simulink model "f_Madgwick"  (R2015a)
settings: Solver=ode4  StartTime=0.0  StopTime=t(len)  FixedStep=1/freq  RelTol=1e-3
InitFcn:
  | clear all
  | clc
  | 
  | RAW = dlmread('manual_6_raw_16-12.txt');
  | 
  | acc = 1/1000*[RAW(:,1) RAW(:,2) RAW(:,3)]';
  | gyro = 1/1000*[RAW(:,4) RAW(:,5) RAW(:,6)]';
  | mag = [RAW(:,7) RAW(:,8) RAW(:,9)]';
  | 
  | freq = 50; %[Hz] Sampling frequency
  | len = length(RAW);
  | 
  | t = 0 : 1/freq : (len-1)/freq;
StopFcn:
  | close all
  | clc
  | %%
  | 
  | Rm = yout(:,1);
  | Pm = yout(:,2);
  | Ym = yout(:,3);
  | 
  | Rq = yout(:,4);
  | Pq = yout(:,5);
  | Yq = yout(:,6);
  | 
  | Rmu = unwrap(Rm);
  | Pmu = unwrap(Pm);
  | Ymu = unwrap(Ym);
  | 
  | Rqu = unwrap(Rq);
  | Pqu = unwrap(Pq);
  | Yqu = unwrap(Yq);
  | 
  | %% Plotting Roll, Pitch and Yaw angles
  | 
  | figure
  | subplot(3,1,1)
  | plot(tout,Rmu, tout, Rqu)
  | title('Roll')
  | ylabel('[deg]')
  | xlabel('[sec]')
  | legend('Rmu','Rqu')
  | subplot(3,1,2)
  | plot(tout,Pmu, tout, Pqu)
  | title('Pitch')
  | ylabel('[deg]')
  | xlabel('[sec]')
  | legend('Pmu','Pqu')
  | subplot(3,1,3)
  | plot(tout,Ymu, tout, Yqu)
  | title('Yaw')
  | ylabel('[deg]')
  | xlabel('[sec]')
  | legend('Ymu','Yqu')
libraries: aerolibutil x2, aerolibtransform2 x2, dspmathops x1
settings Model: CovSFcnEnable=off  Creator=Mattia  LastModifiedBy=pela
settings DataIOCC: ExternalInput=[t u]
settings DebuggingCC: SolverPrmCheckMsg=warning

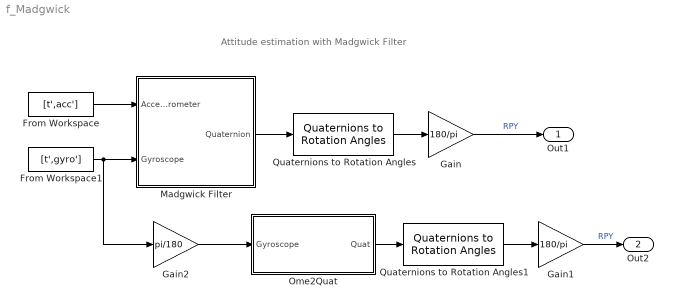
== system f_Madgwick ==
  note: Attitude estimation with Madgwick Filter
  From Workspace : FromWorkspace  VariableName=[t',acc']  SampleTime=0  OutputAfterFinalValue=Setting to zero
  From Workspace1 : FromWorkspace  VariableName=[t',gyro']  SampleTime=0  OutputAfterFinalValue=Setting to zero
  Gain : Gain  Gain=180/pi
  Gain1 : Gain  Gain=180/pi
  Gain2 : Gain  Gain=pi/180
  Madgwick Filter : Subsystem  mask{QUAT0_MF=[1 0 0 0]', beta=0*0.001}
      mask prompts: QUAT0_MF "Quaternion initial condition"; beta "Filter gain"
      mask Display:
      | port_label('input', 1, 'Accelerometer')
      | port_label('input', 2, 'Gyroscope')
      | port_label('Output', 1, 'Quaternion')
  Ome2Quat : Subsystem  mask{QUAT_0=[1 0 0 0]'}
      mask prompts: QUAT_0 "Initial quaternion"
      mask DialogControl DescTextVar Prompt: Here you can set the initial condition for the quaternion integration.
      mask Display:
      | port_label('input', 1, 'Gyroscope')
      | port_label('output', 1, 'Quaternion')
  Quaternions to Rotation Angles : aerolibtransform2/Quaternions to Rotation Angles  rotationOrder=XYZ
  Quaternions to Rotation Angles1 : aerolibtransform2/Quaternions to Rotation Angles  rotationOrder=XYZ
  Out1 : Outport
  Out2 : Outport  Port=2
  wires:
  Quaternions to Rotation Angles/1 -> Gain/1
  Madgwick Filter/1(Quaternion) -> Quaternions to Rotation Angles/1
  From Workspace/1 -> Madgwick Filter/1(Accelerometer)
  Gain/1 -> Out1/1  "RPY"
  Quaternions to Rotation Angles1/1 -> Gain1/1
  Ome2Quat/1(Quat) -> Quaternions to Rotation Angles1/1
  Gain1/1 -> Out2/1  "RPY"
  Gain2/1 -> Ome2Quat/1("Gyroscope ")
  From Workspace1/1 -> Madgwick Filter/2(Gyroscope), Gain2/1

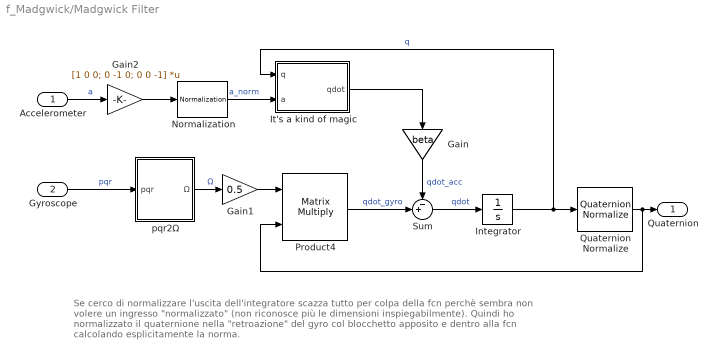
== system f_Madgwick/Madgwick Filter ==
  note: Se cerco di normalizzare l'uscita dell'integratore scazza tutto per colpa della fcn perchè sembra non volere un
      | ingresso "normalizzato" (non riconosce più le dimensioni inspiegabilmente).
      | Quindi ho normalizzato il quaternione nella "retroazione" del gyro col blocchetto apposito e dentro alla fcn calcolando
      | esplicitamente la norma.
  Accelerometer : Inport
  Gyroscope : Inport  Port=2
  Gain : Gain  Gain=beta
  Gain1 : Gain  Gain=0.5
  Gain2 : Gain  Gain=[1 0 0; 0 -1 0; 0 0 -1]  Multiplication=Matrix(K*u)
  Integrator : Integrator  InitialCondition=QUAT0_MF
  It's a kind of magic : MATLAB Function  TreatAsAtomicUnit=on
  Normalization : dspmathops/Normalization  NormType=2-norm  Bias=1e-10  NormOver=Each column  ColComp=on  Dimension=1  outputDataTypeStr=Inherit: Same as product output  outputLastDataTypeStr=Inherit: Same as product output  outputMin=[]  outputMax=[]  accumDataTypeStr=Inherit: Same as product output  accumLastDataTypeStr=Inherit: Same as product output  roundingMode=Floor  overflowMode=off
  Product4 : Product  Multiplication=Matrix(*)
  Quaternion Normalize : aerolibutil/Quaternion Normalize
  Sum : Sum  Inputs=-+|
  pqr2Ω : Subsystem
  Quaternion : Outport
  wires:
  Gyroscope/1 -> pqr2Ω/1(" pqr")  "pqr"
  Gain1/1 -> Product4/1
  pqr2Ω/1(Ω) -> Gain1/1  "Ω"
  Quaternion Normalize/1 -> Quaternion/1, Product4/2
  It's a kind of magic/1(qdot) -> Gain/1
  Normalization/1 -> It's a kind of magic/2(a)  "a_norm"
  Sum/1 -> Integrator/1  "qdot"
  Product4/1 -> Sum/2  "qdot_gyro"
  Integrator/1 -> Quaternion Normalize/1, It's a kind of magic/1(q)  "q"
  Gain/1 -> Sum/1  "qdot_acc"
  Accelerometer/1 -> Gain2/1  "a"
  Gain2/1 -> Normalization/1

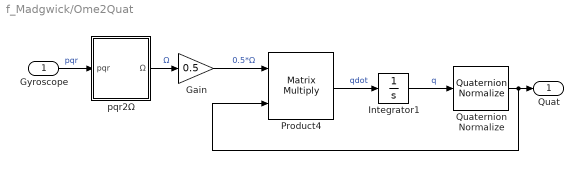
== system f_Madgwick/Ome2Quat ==
  "Gyroscope " : Inport
  Gain : Gain  Gain=0.5
  Integrator1 : Integrator  InitialCondition=QUAT_0
  Product4 : Product  Multiplication=Matrix(*)
  Quaternion Normalize : aerolibutil/Quaternion Normalize
  pqr2Ω : Subsystem
  Quat : Outport
  wires:
  pqr2Ω/1(Ω) -> Gain/1  "Ω"
  Gain/1 -> Product4/1  "0.5*Ω"
  Product4/1 -> Integrator1/1  "qdot"
  "Gyroscope "/1 -> pqr2Ω/1(" pqr")  "pqr"
  Quaternion Normalize/1 -> Product4/2, Quat/1
  Integrator1/1 -> Quaternion Normalize/1  "q"

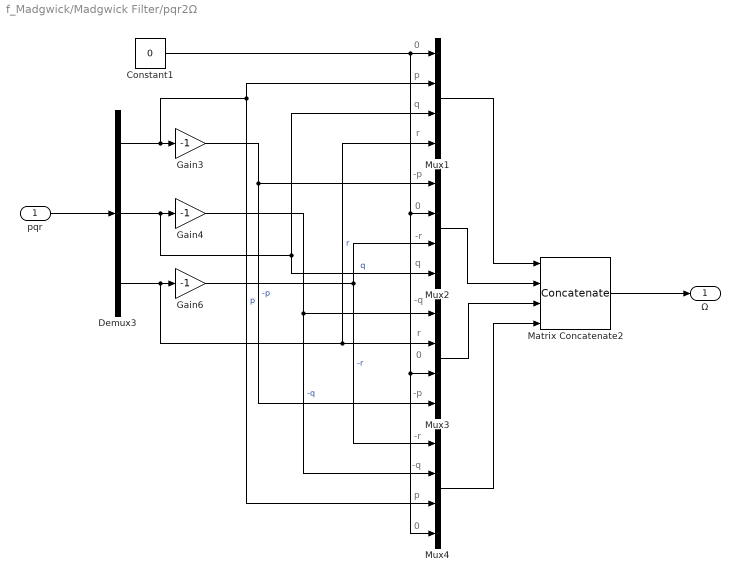
== system f_Madgwick/Madgwick Filter/pqr2Ω ==
  note: 0
  note: p
  note: q
  note: r
  note: -p
  note: 0
  note: -r
  note: q
  note: -q
  note: r
  note: 0
  note: -p
  note: -r
  note: -q
  note: p
  note: 0
  " pqr" : Inport
  Constant1 : Constant  Value=0
  Demux3 : Demux  Outputs=3
  Gain3 : Gain  Gain=-1
  Gain4 : Gain  Gain=-1
  Gain6 : Gain  Gain=-1
  Matrix Concatenate2 : Concatenate  NumInputs=4  Mode=Multidimensional array  ConcatenateDimension=2
  Mux{1..4} (4 alike) : Mux
  Ω : Outport
  wires:
  Gain6/1 -> Mux2/3, Mux4/1  "-r"
  Gain4/1 -> Mux3/1, Mux4/2  "-q"
  Gain3/1 -> Mux2/1, Mux3/4  "-p"
  Demux3/3 -> Gain6/1, Mux1/4, Mux3/2  "r"
  Demux3/2 -> Gain4/1, Mux1/3, Mux2/4  "q"
  Demux3/1 -> Gain3/1, Mux1/2, Mux4/3  "p"
  Matrix Concatenate2/1 -> Ω/1
  Constant1/1 -> Mux1/1, Mux4/4, Mux3/3, Mux2/2
  Mux4/1 -> Matrix Concatenate2/4
  Mux3/1 -> Matrix Concatenate2/3
  Mux2/1 -> Matrix Concatenate2/2
  Mux1/1 -> Matrix Concatenate2/1
  " pqr"/1 -> Demux3/1

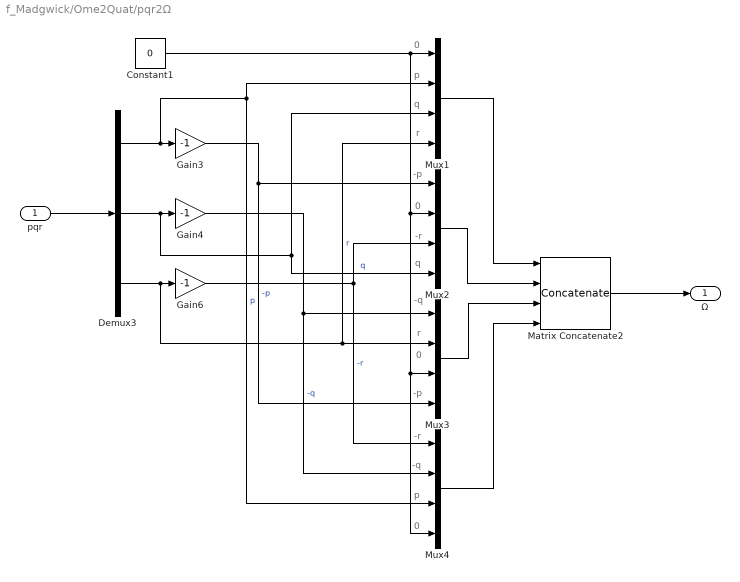
== system f_Madgwick/Ome2Quat/pqr2Ω ==
  note: 0
  note: p
  note: -q
  note: -r
  note: -p
  note: 0
  note: r
  note: -q
  note: q
  note: -r
  note: 0
  note: -p
  note: r
  note: q
  note: p
  note: 0
  " pqr" : Inport
  Constant1 : Constant  Value=0
  Demux3 : Demux  Outputs=3
  Gain3 : Gain  Gain=-1
  Gain4 : Gain  Gain=-1
  Gain6 : Gain  Gain=-1
  Matrix Concatenate2 : Concatenate  NumInputs=4  Mode=Multidimensional array  ConcatenateDimension=2
  Mux{1..4} (4 alike) : Mux
  Ω : Outport
  wires:
  " pqr"/1 -> Demux3/1
  Mux1/1 -> Matrix Concatenate2/1
  Mux2/1 -> Matrix Concatenate2/2
  Mux3/1 -> Matrix Concatenate2/3
  Mux4/1 -> Matrix Concatenate2/4
  Constant1/1 -> Mux2/2, Mux3/3, Mux4/4, Mux1/1
  Matrix Concatenate2/1 -> Ω/1
  Demux3/1 -> Mux4/3, Mux1/2, Gain3/1  "p"
  Demux3/2 -> Mux2/4, Mux1/3, Gain4/1  "q"
  Demux3/3 -> Mux3/2, Mux1/4, Gain6/1  "r"
  Gain3/1 -> Mux3/4, Mux2/1  "-p"
  Gain4/1 -> Mux4/2, Mux3/1  "-q"
  Gain6/1 -> Mux4/1, Mux2/3  "-r"

== matlab function f_Madgwick/Madgwick Filter/It's a kind of magic ==
  data: q input; a input; qdot output
function qdot = GradDesc(q,a)
 % Gradient descent algorithm corrective step
 qnorm = sqrt(q(1)*q(1) + q(2)*q(2) + q(3)*q(3) + q(4)*q(4));
 
 q0 = q(1)/qnorm;
 q1 = q(2)/qnorm;
 q2 = q(3)/qnorm;
 q3 = q(4)/qnorm;
 q0q0 = q0*q0;
 q1q1 = q1*q1;
 q2q2 = q2*q2;
 q3q3 = q3*q3;
 
 ax = a(1);
 ay = a(2);
 az = a(3);
 
 s0 = 4*q0*q2q2 + 2*q2*ax + 4*q0*q1q1 - 2*q1*ay;
 s1 = 4*q1*q3q3 - 2*q3*ax + 4*q0q0*q1 - 2*q0*ay - 4*q1 + 8*q1*q1q1 + 8*q1*q2q2 + 4*q1*az;
 s2 = 4*q0q0*q2 + 2*q0*ax + 4*q2*q3q3 - 2*q3*ay - 4*q2 + 8*q2*q1q1 + 8*q2*q2q2 + 4*q2*az;
 s3 = 4*q1q1*q3 - 2*q1*ax + 4*q2q2*q3 - 2*q2*ay;

 snorm = sqrt(s0*s0 + s1*s1 + s2*s2 + s3*s3);
 
 s0 = s0/snorm;
 s1 = s1/snorm;
 s2 = s2/snorm;
 s3 = s3/snorm;
 
qdot = [s0 s1 s2 s3]';
